simulink model "FD_THRUSTER"  (R2019b)
settings: Solver=FixedStepAuto  StartTime=0.0  StopTime=10.0  RelTol=1e-3
undefined symbols (not defined in the file): w_static
settings Model: Creator=lbend  LastModifiedBy=lbend
settings DebuggingCC: UnconnectedInputMsg=none  UnconnectedOutputMsg=none  UnconnectedLineMsg=none  SFMachineParentedDataDiag=error
settings ModelReferenceCC: EnableRefExpFcnMdlSchedulingChecks=off
settings RTWCC: Description=Generic Real-Time Target

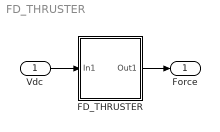
== system FD_THRUSTER ==
  Vdc : Inport
  FD_THRUSTER : Subsystem
  Force : Outport
  wires:
  Vdc/1 -> FD_THRUSTER/1(In1)
  FD_THRUSTER/1(Out1) -> Force/1

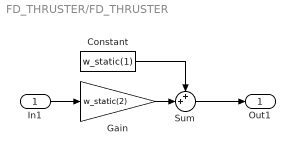
== system FD_THRUSTER/FD_THRUSTER ==
  In1 : Inport
  Constant : Constant  Value=w_static(1)
  Gain : Gain  Gain=w_static(2)
  Sum : Sum  Inputs=++|
  Out1 : Outport
  wires:
  Constant/1 -> Sum/1
  Gain/1 -> Sum/2
  In1/1 -> Gain/1
  Sum/1 -> Out1/1
